simulink model "gridMapModel"  (R2014a)
settings: Solver=ode45  StartTime=0.0  StopTime=Inf  RelTol=1e-3
InitFcn:
  | close all;
  | 
  | lid = LIDAR();
  | rob = DifferentialRobot();
  | rob.dt = 0.02;
  | rob.attachLidar(lid, [0.6,0,0]);
  | 
  | subplot(1, 2, 1);
  | gm = GridMap([40 40], 0.1);
  | ghMap = imshow(gm.map);
  | 
  | 
  | ghPlot =subplot(1, 2, 2);
  | hold on;
  | axis equal;
  | hold on;
  | whitebg([0 0 0]);
  | grid on;
  | pl = Plotter(ghPlot);
libraries: iWalkerLib x1
settings Model: Creator=Brian  LastModifiedBy=Brian

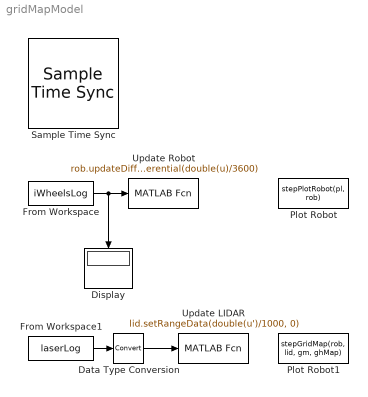
== system gridMapModel ==
  Data Type Conversion : DataTypeConversion
  Display : Display
  From Workspace : FromWorkspace  VariableName=iWheelsLog  SampleTime=0.01  Interpolate=off  OutputAfterFinalValue=Setting to zero
  From Workspace1 : FromWorkspace  VariableName=laserLog  SampleTime=0.3  Interpolate=off  OutputAfterFinalValue=Setting to zero
  Plot Robot : MATLABFcn  MATLABFcn=stepPlotRobot(pl, rob)  OutputDimensions=0  SampleTime=1/25
  Plot Robot1 : MATLABFcn  MATLABFcn=stepGridMap(rob, lid, gm, ghMap)  OutputDimensions=0  SampleTime=1
  Sample Time Sync : iWalkerLib/Sample Time Sync  Priority=8  SampleTime=0.01
  Update LIDAR : MATLABFcn  MATLABFcn=lid.setRangeData(double(u')/1000, 0)  OutputDimensions=0
  Update Robot : MATLABFcn  MATLABFcn=rob.updateDifferential(double(u)/3600)  OutputDimensions=0
  wires:
  From Workspace/1 -> Update Robot/1, Display/1
  From Workspace1/1 -> Data Type Conversion/1
  Data Type Conversion/1 -> Update LIDAR/1
